simulink model "dspstfft_audio_V2_2015a"  (R2015a)
settings: Solver=FixedStepDiscrete  StartTime=0.0  StopTime=inf  RelTol=1e-3
model workspace: external: MAT-File mtlb.mat (data not in the file)
undefined symbols (not defined in the file or in its folder): jet
libraries: dspsnks4 x2, dspsrcs4 x1, dspmisc x1, dspspect3 x1, dspmathops x1
settings Model: CovMetricSettings=d  ExtModeAutoUpdateStatusClock=off  Creator=The MathWorks Inc.  LastModifiedBy=子皓
settings DataIOCC: SignalLoggingSaveFormat=ModelDataLogs  SaveOutput=off  SaveTime=off  SignalLoggingName=logsOut
settings OptimizationCC: BlockReduction=off  BooleanDataType=off  ExpressionDepthLimit=2147483647  InitFltsAndDblsToZero=on
settings DebuggingCC: SaveWithParameterizedLinksMsg=none  UnderspecifiedInitializationDetection=Classic  MergeDetectMultiDrivingBlocksExec=none  SignalResolutionControl=TryResolveAllWithWarning  MultiTaskDSMMsg=warning  MultiTaskCondExecSysMsg=none  FcnCallInpInsideContextMsg=UseLocalSettings  StateNameClashWarn=warning
settings HardwareCC: ProdHWDeviceType=Specified
settings GRTTargetCC: TargetFcnLib=ansi_tfl_tmw.mat  CombineOutputUpdateFcns=off  GRTInterface=on

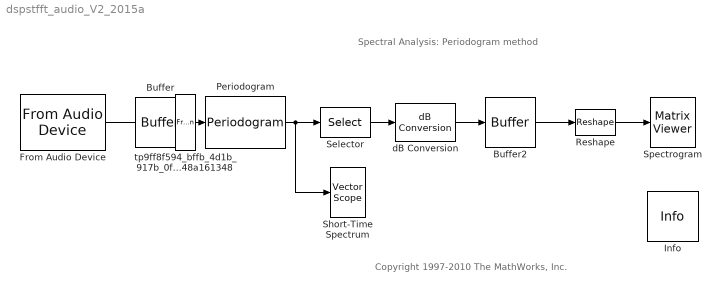
== system dspstfft_audio_V2_2015a ==
  note: Spectral Analysis: Periodogram method
  note: Copyright 1997-2010 The MathWorks, Inc.
  Buffer : Buffer  N=128  V=48  TreatMby1Signals=One channel
  Buffer2 : Buffer  N=48*64  V=46*64  ic=-70  TreatMby1Signals=One channel
  From Audio Device : dspsrcs4/From Audio Device  deviceName=Default  numChannels=1  sampleRate=44100  deviceDatatype=Determine from output data type  autoBufferSize=on  bufferSize=4096  queueDuration=1.0  frameSize=80  outputDatatype=double  defaultInputChannelMapping=on  inputChannelMapping=1:2  outputNumOverrunSamples=off
  Info : dspmisc/Info  SystemSampleTime=-1
  Periodogram : dspspect3/Periodogram  measurement=Power spectral density  wintype=Hamming  Rs=50  beta=5  winsamp=Periodic  FFTImplementation=Auto  inheritFFT=on  fftsize=128  navg=2  inheritTs=on  Ts=1
  Reshape : Reshape  OutputDimensionality=Customize  OutputDimensions=[64 48]
  Selector : Selector  InputPortWidth=128  IndexOptions=Index vector (dialog)  Indices=1:64  OutputSizes=1
  Short-Time Spectrum : dspsnks4/Vector Scope  ScopeProperties=on  Domain=Frequency  HorizSpan=1  DisplayProperties=off  AxisGrid=on  Memory=off  FrameNumber=off  AxisLegend=off  AxisZoom=off  OpenScopeAtSimStart=on  OpenScopeImmediately=off  FigPos=[50 50 380 320]  AxisProperties=off  XUnits=Hertz  XRange=[0...Fs/2]  InheritXIncr=off  XIncr=1/8000  XLabel=Samples  XLimit=Auto  XMin=0  XMax=1  XStart=0  YUnits=dB  YLabel=Magnitude, dB  LineProperties=off  XAxisParamsVer=6.9
      settings: YMin=-95  YMax=-30
  Spectrogram : dspsnks4/Matrix Viewer  ImageParams=off  CMapStr=jet(256)  AxisColorbar=on  AxisParams=off  AxisOrigin=Lower left corner  XLabel=Time Index  YLabel=Frequency Index  ZLabel=dB Magnitude  FigPos=[550 50 380 320]  AxisZoom=off
      settings: YMin=-150  YMax=-65
  dB Conversion : dspmathops/dB Conversion  dBtype=dB  intype=Amplitude  R=1  fuzz=on
  tp9ff8f594_bffb_4d1b_917b_0f448a161348 : FrameConversion  InheritSamplingMode=off  OutFrame=Sample-based
  wires:
  Buffer/1 -> Periodogram/1
  Selector/1 -> dB Conversion/1
  Periodogram/1 -> Short-Time Spectrum/1, Selector/1
  Buffer2/1 -> Reshape/1
  Reshape/1 -> Spectrogram/1
  dB Conversion/1 -> Buffer2/1
  From Audio Device/1 -> tp9ff8f594_bffb_4d1b_917b_0f448a161348/1
  tp9ff8f594_bffb_4d1b_917b_0f448a161348/1 -> Buffer/1
